simulink model "AdaptiveFilter"  (R2022b)
settings: Solver=VariableStepAuto  StartTime=0.0  StopTime=inf  RelTol=1e-3
model workspace (MAT data in the model file):
  a_1 = 3.55071544647
  a_2 = 1
  b_1 = Simulink.Parameter
  b_1.Value = 1
  b_1.DataType = 'auto'
  b_1.Complexity = 'real'
  b_1.Dimensions = [1 1]
  b_2 = Simulink.Parameter
  b_2.Value = 1
  b_2.DataType = 'auto'
  b_2.Complexity = 'real'
  b_2.Dimensions = [1 1]
  b_3 = Simulink.Parameter
  b_3.Value = 1
  b_3.DataType = 'auto'
  b_3.Complexity = 'real'
  b_3.Dimensions = [1 1]
settings Model: Creator=Ceribro  LastModifiedBy=Ceribro

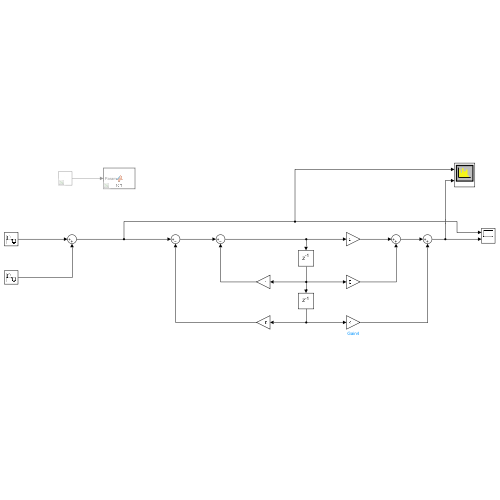
[thumbnail: Simulink's stored preview of the top-level diagram]
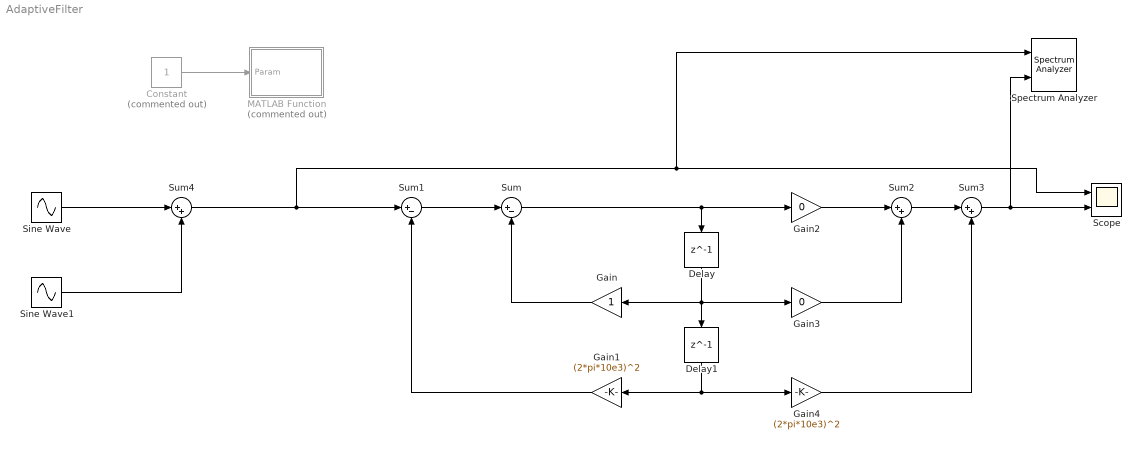
== system AdaptiveFilter ==
  Constant : Constant  Commented=on
  Delay : Delay  DelayLength=1  InitialCondition=0
  Delay1 : Delay  DelayLength=1  InitialCondition=0
  Gain : Gain
  Gain1 : Gain  Gain=(2*pi*10e3)^2
  Gain2 : Gain  Gain=0
  Gain3 : Gain  Gain=0
  Gain4 : Gain  Gain=(2*pi*10e3)^2
  MATLAB Function : MATLAB Function  Commented=on  TreatAsAtomicUnit=on
  Scope : Scope  NumInputPorts=2
  Sine Wave : Sin  Frequency=1000*2*pi  SampleTime=1/44.1e3
  Sine Wave1 : Sin  Frequency=15000*2*pi  SampleTime=1/44.1e3
  Spectrum Analyzer : SpectrumAnalyzer  NumInputPorts=2
  Sum : Sum  Inputs=|+-
  Sum1 : Sum  Inputs=|+-
  Sum2 : Sum  Inputs=|++
  Sum3 : Sum  Inputs=|++
  Sum4 : Sum  Inputs=|++
  wires:
  Delay/1 -> Gain3/1, Gain/1, Delay1/1
  Delay1/1 -> Gain4/1, Gain1/1
  Sum1/1 -> Sum/1
  Sum/1 -> Gain2/1, Delay/1
  Gain/1 -> Sum/2
  Gain1/1 -> Sum1/2
  Gain2/1 -> Sum2/1
  Gain3/1 -> Sum2/2
  Gain4/1 -> Sum3/2
  Sum2/1 -> Sum3/1
  Sum4/1 -> Sum1/1, Spectrum Analyzer/1, Scope/1
  Sum3/1 -> Spectrum Analyzer/2, Scope/2
  Constant/1 -> MATLAB Function/1(Param)
  Sine Wave1/1 -> Sum4/2
  Sine Wave/1 -> Sum4/1

== matlab function AdaptiveFilter/MATLAB Function ==
  data: Param input
function fcn(Param)
set_param('AdaptiveFilter','a_1',int2str( Param ));
